simulink model "stewart_platform_final3"  (R2017a)
settings: Solver=ode45  StartTime=0.0  StopTime=40  MaxStep=0.2  RelTol=1e-3  EnableMultiTasking=on
model workspace (MAT data in the model file):
  g_density = 5
undefined symbols (not defined in the file): B, nom_length, P, X, Y, Z
libraries: nesl_utility x13, sm_stewart_platform_lib x8, sm_lib x7
(part 1 of 2)
Description:
  | Stewart Platform
  | 
  | This model shows a Stewart platform manipulator that can track a
  | parameterized reference trajectory. The shape, size, and kinematics of
  | the manipulator are highly configurable.
  | 
  | The reference trajectory is
  | specified in 6-D pose space, and an inverse kinematics module
  | converts it into one through 6-D leg position space.  A generic PID
  | controller attempts to drive the manipulator along the desired
  | trajectory.
  | 
  | 
  | Copyright 2011-2017 The MathWorks, Inc.
settings Model: FPTRunName=Active  Creator=MathWorks  LastModifiedBy=Omar
settings DataIOCC: LimitDataPoints=on  SaveFormat=Array  SignalLoggingSaveFormat=ModelDataLogs
settings OptimizationCC: ExpressionDepthLimit=2147483647  LifeSpan=inf
settings DebuggingCC: UnderspecifiedInitializationDetection=Classic  MergeDetectMultiDrivingBlocksExec=none  SolverPrmCheckMsg=warning  FcnCallInpInsideContextMsg=warning  StateNameClashWarn=warning  SFUnexpectedBacktrackingDiag=warning  SFNoUnconditionalDefaultTransitionDiag=warning  SFExecutionAtInitializationDiag=none
settings HardwareCC: ProdBitPerPointer=32  ProdBitPerSizeT=32  ProdBitPerPtrDiffT=32  ProdLargestAtomicFloat=None  ProdIntDivRoundTo=Undefined  ProdEndianess=Unspecified  ProdWordSize=32  ProdHWDeviceType=32-bit Generic
settings ModelReferenceCC: PropagateSignalLabelsOutOfModel=off
settings GRTTargetCC: TargetLangStandard=C89/C90 (ANSI)  GeneratePreprocessorConditionals=Disable all  CombineOutputUpdateFcns=off  GRTInterface=on
settings ConfigComp: CovMetricSettings=dw  CovHtmlReporting=on  CovSaveCumulativeToWorkspaceVar=on  CovSaveSingleToWorkspaceVar=on  CovExternalEMLEnable=off
settings SimscapeCC: SimscapeLogDataHistory=15000
settings ConfigurationSet: Description=SimMechanics 2G

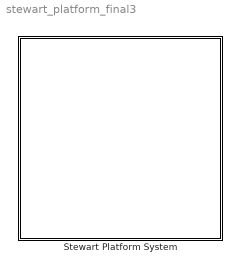
== system stewart_platform_final3 ==
  Stewart Platform System : Subsystem  mask(Stewart Platform System){base_rad=28, base_thick=8, platform_rad=18, platform_thick=2, hex_skew=-0.25, upper_leg_len=10, lower_leg_len=14, leg_rad=3, collar_thick=0.5, gripper_height=30, claw_length=8, claw_width=3, claw_thick=1, end_eff_base_thick=2, flange_len=3, flange_width=2.25, flange_thick=.8, ic_R=eye(3), ic_d=[0 0 71]', Kp=300, Ki=20, Kd=5}
      mask prompts: base_rad "Base Radius  (cm)"; base_thick "Base Thickness (cm)"; platform_rad "Platform Radius (cm)"; platform_thick "Platform Thickness (cm)"; hex_skew "Hexagon Skew"; upper_leg_len "Upper Leg Length (cm)"; lower_leg_len "Lower Leg Length (cm)"; leg_rad "Leg Radius (cm)"; collar_thick "Collar Thickness (cm)"; gripper_height "Gripper Height (cm)"; claw_length "Claw Length (cm)"; claw_width "Claw Width (cm)"; claw_thick "Claw Thickness (cm)"; end_eff_base_thick "Base Thickness (cm)"; flange_len "Flange Length (cm)"; flange_width "Flange Width (cm)"; flange_thick "Flange Thickness (cm)"; ic_R "Rotation Matrix [3 x 3]"; ic_d "Displacement Vector (cm) [3 x 1]"; Kp "Controller Proportional Gain (N / cm)"; Ki "Controller Integral Gain (N / (cm s))"; Kd "Controller Derivative Gain (N / (cm / s)))"
      mask help:
      | Models a complete Stewart platform manipulator system.  The system can be driven to position and orient a special gripper frame according to specified trajectories.
      |
      | The system comprises a mechanical manipulator, an inverse kinematics module, and a control system.
      mask init:
      | params = struct( ...
      |     'base_thick',        base_thick,     ...
      |     'base_radius',       base_rad,       ...
      |     'platform_thick',    platform_thick, ...
      |     'platform_radius',   platform_rad,   ...
      |     'skew',              hex_skew,       ...
      |     'flange_length',     flange_len,     ...
      |     'flange_width',      flange_width,   ...
      |     'flange_thick',      flange_thick,   ...
      |     'leg_radius',        leg_rad,        ...
      |     'upper_leg_length',  upper_leg_len,  ...
      |     'lower_leg_length',  lower_leg_len,  ...
      |     'gripper_height',    gripper_height  ...
      |     );
      | 
      | [B, P, nom_length] = sm_stewart_platform_setup(params);
      | 
      | lengths = sm_stewart_platform_ik(B, P, nom_length, ic_R, ic_d);
      mask Help:
      | A <em>Stewart Platform System</em> models a complete Stewart platform manipulator system.  The system can be driven to position and orient a special gripper frame according to specified trajectories.
      | 
      | <h3>Subsystems</h3>
      | 
      | A Stewart platform system comprises three primary subsystems:
      | 
      | <ol>
      | 
      | <li><b>Manipulator</b> The manipulator is the Simscape Multibody subsystem describing the mechanical structure of the Stewart platform.  The manipulator contains two hexagonal plates, a lower base plate and an upper platform plate, connected by six articulated legs.  The base plate is anchored to the world frame, and the platform plate is controlled to position and orient the gripper frame. The manipulator component provides sensing and actuation signals to interface to a controller.
      | 
      |   The manipulator is highly parameterized.  Most parameters of the Stewart platform system are physical lengths and other parameters that control the shapes and sizes of the components of the manipulator. By varying these parameters, a wide range of Stewart platform manipulators can be realized.
      | 
      | <li><b>Inverse Kinematics (IK) Module</b> The inverse kinematics module is a pure Simulink subsystem that maps time-varying signals describing the desired position and orientation of the gripper frame into time-varying scalar signals specifying the positions and velocities of the prismatic primitives of the leg joints.  This is an essential component of a complete Stewart platform system because the user of the system typically expresses a desired trajectory in the 6-D space of positions and orientations of the gripper frame, but the manipulator control is simplest in the 6-D space of leg joint positions. The IK module forms the bridge between these two spaces.
      | 
      |   The mathematics performed within the IK module is heavily dependent on the physical parameters that determine the shape and size of the manipulator itself.  Most of the parameters that govern the manipulator are also used within the IK module.
      | 
      | <li><b>Control System</b> The control system is a pure Simulink subsystem that attempts to drive the gripper frame along its desired trajectory by controlling the positions of the prismatic primitives of the leg joints. It uses a standard PID control scheme, with gains specified by Stewart platform system parameters.  The control uses no information about the forward or inverse kinematics of the platform; it simply tries to drive a point along a trajectory in 6-D space.
      | 
      |   The controller takes both the desired and actual leg position vectors and the first derivatives of these quantities.  It generates a 6-D commanded force output that can be used to drive the six leg lengths to thei desired values.
      | 
      |   Because the size and shape of the Stewart platform manipulator can vary significantly depending on the parameter settings, the controller gains may need to be adjusted in order to control the manipulator to the desired trajectory.
      | 
      | </ol>
      | 
      | <h3>Base and Platform Plates</h3>
      | 
      | The <em>Plates</em> tab parameters specify the geometry of the base and platform hexagon plates of the Stewart platform manipulator.  See the documentation of the <em>Hexagon Plate</em> library block for details.
      | 
      | <ul>
      | 
      | <li> <b>Base Radius</b> The radius of the base plate.  The vertices of the hexagonal cross section all lie on a circle of this radius.
      | 
      | <li> <b>Base Thickness</b> The thickness of the base plate.
      | 
      | <li> <b>Platform Radius</b> The radius of the platform plate.  The vertices of the hexagonal cross section all lie on a circle of this radius.
      | 
      | <li> <b>Platform Thickness</b> The thickness of the platform plate.
      | 
      | <li> <b>Hexagon Skew</b> The common skew factor of the base and platform plates. This value, in the range (-0.5, +0.5), determines the shape of the three-fold symmetric hexagons.  A zero skew factor produces regular hexagons.  As the skew factor magnitude increases, the hexagons become more triangular.
      | 
      | </ul>
      | 
      | <h3>Legs</h3>
      | 
      | The <em>Legs</em> tab parameters specify the common geometry of the six legs of the Stewart platform manipulator.  See the documentation of the <em>Leg</em> library block for details.
      | 
      | <ul>
      | 
      | <li> <b>Upper Leg Length</b> The length of the upper leg, including its end collars.
      | 
      | <li> <b>Lower Leg Length</b> The length of the lower leg, including its end collars.
      | 
      | <li> <b>Leg Radius</b> The common radius of the upper and lower leg segments. Each segment's cross section is a regular hexagon inscribed in a circle of this radius.
      | 
      | <li> <b>Collar Thickness</b> The thickness of the hexagonal collars adjoined to the ends of each leg segment.
      | 
      | </ul>
      | 
      | <h3>End Effector</h3>
      | 
      | The <em>End Eff</em> tab parameters specify the geometry of the end effector attached to the platform plate of the Stewart platform manipulator. See the documentation of the <em>End Effector</em> block within the <em>Manipulator</em> subsystem for details.
      | 
      | <ul>
      | 
      | <li> <b>Gripper Height</b> The vertical distance from the origin of the gripper frame to the top surface of the movable platform plate.
      | 
      | <li> <b>Claw Length</b> The length (height) of the trapezoidal claws of the gripper.
      | 
      | <li> <b>Claw Width</b> The width of the trapezoidal claws of the gripper where they attach to the gripper base.
      | 
      | <li> <b>Claw Thickness</b> The thickness of the trapezoidal claws of the gripper.
      | 
      | <li> <b>Base Thickness</b> The thickness of the triangular gripper base.
      | 
      | </ul>
      | 
      | <h3>Flanges</h3>
      | 
      | The <em>Flanges</em> tab parameters specify the common geometry of the 48 flanges attached to the hexagonal plates and legs of the Stewart platform manipulator.  Each of the 12 universal joints is supported by four flanges.  See the documentation of the <em>Flange</em> library block for details.
      | 
      | <ul>
      | 
      | <li> <b>Flange Length</b> The length of the rectangular prism portion of the flanges.
      | 
      | <li> <b>Flange Width</b> The width of the rectangular prism portion of the flanges.
      | 
      | <li> <b>Flange Thickness</b> The thickness of the flanges.
      | 
      | </ul>
      | 
      | <h3>Initial Conditions</h3>
      | 
      | The <em>IC</em> tab parameters specify the initial conditions of the Stewart Platform manipulator for simulation.  Specifically, these specify the <em>position</em> of the manipulator; the simulation always starts from a rest (zero velocity) state.
      | 
      | The initial position is defined by specifying pose of the gripper frame relative to the world frame.  This is typically a convenient parameterization for a user of the manipulator.  The world frame is also the reference frame of the manipulator base plate.  This is a frame with origin at the center of the manipulator base (which is in its interior), and with z-axis pointed directly upward.
      | 
      | An Update Diagram (Ctrl-D) operation will attempt to assemble the manipulator in the specified initial position.  Some initial positions may be incompatible with the kinematics of the manipulator, based on other parameter settings.  In such cases, the assembly will fail.
      | 
      | Also note that if the initial position differs significantly from the desired trajectory (specified through the input signal ports) at time zero, the manipulator's motion may be subject to large transients at the start of simulation.
      | 
      | <ul>
      | 
      | <li> <b>Rotation Matrix</b> The rotation matrix mapping directions in the gripper frame to directions in the world frame.  This should be a 3 x 3 orthogonal matrix determinant +1.  The columns of this matrix are the canonical i, j, and k unit vectors of the gripper frame resolved in world frame coordinates.
      | 
      | <li> <b>Displacement Vector</b> The location of the origin of the gripper frame in world frame coordinates.  This should be a 3 x 1 column vector.  The z-coordinate should generally be positive, on the order of the nominal lengths of the legs.
      | 
      | </ul>
      | 
      | If the rotation matrix is the identity and the x- and y-coordinates of the displacement vector are zero, the initial configuration of the manipulator will be symmetric with all leg positions equal.
      | 
      | <h3>Controller Gains</h3>
      | 
      | The <em>Control</em> tab parameters specify the gains of the internal controller used to control the manipulator's pose according to a specified trajectory.  The controller uses a generic PID control scheme.  The gains may need to be adjusted to be appropriate if the parameters governing the size and kinematics of the manipulator are changed significantly.
      | 
      | See the documentation of the <em>Controller</em> subsystem for details.
      | 
      | <ul>
      | 
      | <li> <b>Controller Proportional Gain</b> The proportional (P) gain of the internal PID controller.
      | 
      | <li> <b>Controller Integral Gain</b> The integral (I) gain of the internal PID controller.
      | 
      | <li> <b>Controller Derivative Gain</b> The derivative (D) gain of the internal PID controller.
      | 
      | </ul>
      | 
      | 
      | 
      | <h3>Ports</h3>
      | 
      | <ul>
      | 
      | <li><b>d</b> The desired displacement vector of the gripper frame relative to the world frame as a signal input.  This value should be a 3 x 1 vector in units of centimeters.  It specifies the desired origin of the gripper frame in world frame coordinates as a function of time.  This signal is analogous to the <em>Displacement Vector</em> on the <em>IC</em> parameter tab.
      | 
      | <li><b>R</b> The desired rotation matrix from the gripper frame to the world frame as a signal input.  This value should be a 3 x 3 orthogonal matrix with +1 determinant.  The columns of this matrix are the canonical i, j, and k unit vectors of the gripper frame resolved in world frame coordinates, specified as functions of time.  This signal is analogous to the <em>Rotation Matrix</em> on the <em>IC</em> parameter tab.
      | 
      | <li><b>d'</b> The first time derivative of the desired displacement vector of the gripper frame relative to the world frame as a signal input.  This value should be the first time derivative of the signal provided on the <em>d</em> port: a 3 x 1 vector in units of centimeters/second. It specifies the velocity of the origin of the gripper frame in  world frame coordinates as a function of time.
      | 
      | <li><b>R'</b> The first time derivative of the desired rotation matrix from the gripper frame to the world frame as a signal input.  This value should be the first time derivative of the signal provided on the <em>R</em> port: a 3 x 3 matrix.
      | 
      | <li><b>Pos</b> The position of the gripper with respect to the world frame as a 3 x 1 position vector in units of centimeters.
      | </ul>
      | 
      | <!--  LocalWords:  Eff IC Ctrl IK
      |  -->
      mask Display:
      | image(imread('StewPlatBlock.png'))
      | color('yellow')
      | port_label('Input', 1, 'd')
      | port_label('Input', 2, 'R')
      | port_label('Input', 3, 'd''')
      | port_label('Input', 4, 'R''')
      | port_label('Output', 1, 'Pos')

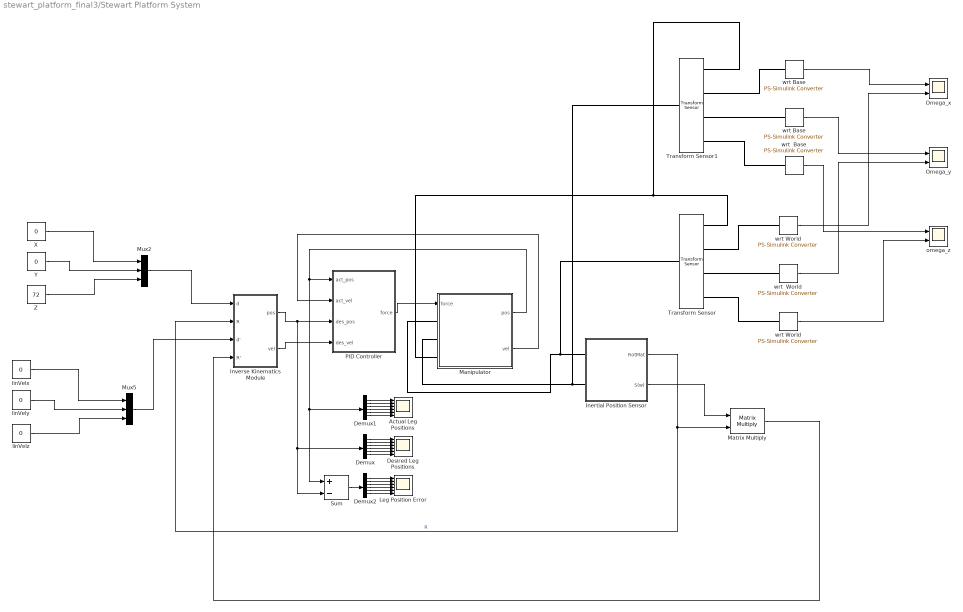
== system stewart_platform_final3/Stewart Platform System ==
  " wrt World" : nesl_utility/PS-Simulink Converter  PhysicalDomain=network_engine_domain  SubClassName=ps_output  LeftPortType=input  RightPortType=output  PseudoPeriodic=off  Frequencies=[]  Unit=1  AffineConversion=off
  Actual Leg Positions : Scope  NumInputPorts=6
  Demux : Demux  Outputs=6
  Demux1 : Demux  Outputs=6
  Demux2 : Demux  Outputs=6
  Desired Leg Positions : Scope  NumInputPorts=6
  Inertial Position Sensor : Subsystem
  Inverse Kinematics Module : Subsystem  mask(Stewart Platform Inverse Kinematics){}
      mask help:
      | Performs the essential inverse kinematic computations for a Stewart platform manipulator.
      |
      | Given a desired dynamic state of a Stewart platform manipulator specified by a 3-D rigid transformation from the gripper frame to the base reference frame, and the first time derivative of this transformation, this block computes the positions and velocities of the prismatic primitives of the six cylindrical leg joints necessary to achieve the desired dynamic state.
      mask Help:
      | A <em>Stewart Platform Inverse Kinematics</em> performs the essential inverse kinematic computations for a Stewart platform manipulator.
      | 
      | Given a desired dynamic state of a Stewart platform manipulator specified by a 3-D rigid transformation from the gripper frame to the base reference frame, and the first time derivative of this transformation, this block computes the positions and velocities of the prismatic primitives of the six cylindrical leg joints necessary to achieve the desired dynamic state.
      | 
      | <h3>Manipulator Transformation</h3>
      | 
      | The desired dynamic state of a Stewart platform manipulator may be specified by a single 3-D rigid transformation, called the <em>manipulator transformation</em>, and its time derivative.  The transformation is from <em>gripper</em> frame to <em>base</em> frame coordinates.  The base frame is attached to the base plate of the manipulator.  Its origin is located at the center of the base, and the z-axis points directly upward.  The gripper frame is located somewhere directly above the center of platform plate of the manipulator, and is aligned with the base frame when the positions of the prismatic primitives of all six cylindrical leg joints are equal.
      | 
      | In the following discussions, let <b>R</b> and <b>d</b> specify the rotation matrix and displacement vector, respectively, of the manipulator transformation. That is, <b>d</b> is the origin of the gripper frame specified in base frame coordinates, and the columns of <b>R</b> are the canonical <b>i</b>, <b>j</b>, and <b>k</b> vectors of the gripper frame resolved in base frame coordinates.
      | Let <b>R'</b> and <b>d'</b> be the first time derivatives of <b>R</b> and <b>d</b>, respectively.
      | 
      | <h3>Inverse Kinematics</h3>
      | 
      | Each of the six legs of the manipulator is attached between a pair of universal joints: one on the base plate and one on the platform plate.  Each leg has an internal knee joint with a sensed and actuated prismatic primitive.
      | Let <em>q_i</em> and <em>q_i'</em> be the position and velocity of this primitive on Leg <em>i</em>.  Let <em>L0</em> denote the <em>nominal</em> lengths of the legs.  This is the length of a leg when its prismatic primitive is at the zero position.
      | 
      | The goal of the inverse kinematics computation is to determine the values of <em>q_i</em> and <em>q_i'</em> for i = 1, ..., 6 needed to achieve a particular manipulator transformation and its derivative.
      | 
      | The key to understanding the inverse kinematics computations is to consider the positions of the centers of the pairs of universal joints.  (These points are the centers of the crosspieces visible in the visualization of the manipulator.)
      | 
      | Let <b>b</b>_i and <b>p</b>_i be the 3-D points specifying the center of the universal joints on the base and platform plates, respectively, to which Leg <em>i</em> is connected. <b>b</b>_i is specified in base frame coordinates, and <b>p</b>_i is specified in gripper frame coordinates.  Then the desired position of the prismatic primitive of the knee joint of Leg <em>i</em> is given by
      | 
      | <em>q_i</em> = || <b>R</b> <b>p</b>_i + <b>d</b> - <b>b</b>_i || - <em>L0</em>.
      | 
      | Denote the vector within the norm expression above as <b>o</b>_i (<b>o</b> for <em>offset</em>).
      | 
      | The desired velocity of the prismatic primitive of the knee joint of Leg <em>i</em> is obtained by differentiating the expression for <em>q_i</em>. Noting that <b>p</b>_i, <b>b</b>_i, and <em>L0</em> are constant, the result is:
      | 
      | <em>q_i'</em> = [ (<b>R'</b> <b>p</b>_i + <b>d'</b>) . <b>o</b>_i ] / || <b>o</b>_i ||.
      | 
      | Note that the denominator of this expression is equal to the vector norm in the expression for <em>q_i</em>.
      | 
      | This block computes the values of all six prismatic primitive positions and velocities according to the expressions above.  The computation of the (constant) <b>p</b>_i and <b>b</b>_i points is highly dependent on the manipulator kinematics and done in the mask initialization of the containing <em>Stewart Platform System</em> block.
      | 
      | <h3>Ports</h3>
      | 
      | <ul>
      | 
      | <li> <b>d</b> The displacement vector of the desired manipulator transformation (see above) in units of centimeters.
      | 
      | <li> <b>R</b> The rotation matrix of the desired manipulator transformation (see above).
      | 
      | <li> <b>d'</b> The time derivative of the displacement vector of the desired manipulator transformation in units of centimeters/second.
      | 
      | <li> <b>R'</b> The time derivative of the rotation matrix of the desired manipulator transformation.
      | 
      | <li> <b>pos</b> The computed positions of the prismatic primitives of the six leg joints, as a 6 x 1 vector in units of centimeters.
      | 
      | <li> <b>vel</b> The computed velocities of the prismatic primitives of the six leg joints, as a 6 x 1 vector in units of centimeters/second.
      | 
      | 
      | </ul>
      | 
      | <!--  LocalWords:  ith pos vel
      |  -->
  Leg Position Error : Scope  NumInputPorts=6
  Manipulator : Subsystem  mask(Stewart Platform Manipulator){}
      mask help: Models the mechanical portion of a complete Stewart platform manipulator system: the manipulator itself. Almost all of the Simscape Multibody blocks of the full system are contained in the manipulator subsystem.
      mask Help:
      | A <em>Stewart Platform Manipulator</em> models the mechanical portion of a complete Stewart platform manipulator system: the manipulator itself.  Almost all of the Simscape Multibody blocks of the full system are contained in the manipulator subsystem.
      | 
      | The manipulator subsystem exposes two frames: the world frame, to which the base is anchored, and the gripper frame, which is the frame at the distil end of the end effector.  Typically, a user wants to control the manipulator transformation, which is the 3-D rigid transformation from the gripper frame to the world frame.
      | 
      | The manipulator subsystem has no internal control.  However, it reports the positions and velocities of the prismatic primitives of all six cylindrical leg joints as output signals and takes the actuation forces to be applied to these primitives as input signals.  When connected to an appropriate controller, these signals are sufficient to provide any of a variety of control schemes for the manipulator.
      | 
      | <h3>Parameterization</h3>
      | 
      | The manipulator is highly parameterized.  Most of the physical dimensions of its component pieces can be controlled via parameters.  These parameters are all defined in the containing <em>Stewart Platform System</em>.  The manipulator's parameters are inherited from that block; they are not defined explicitly in this block's mask.  The parameters are also needed for the <em>Stewart Platform Inverse Kinematics</em> block.
      | 
      | See the documentation of the <em>Stewart Platform System</em> block for details.
      | 
      | <h3>Ports</h3>
      | 
      | <ul>
      | 
      | <li> <b>gripper</b> The gripper frame.  This frame is fixed at the distil end of the end effector attached to the platform plate of the Stewart platform manipulator.  It is identified with a frame glyph in the visualization of the manipulator.  Typically, a user of the manipulator wants to control the pose of this frame, with respect to a reference frame such as world.
      | 
      | <li> <b>world</b> The world frame.  This is also the reference frame of the base plate of the Stewart platform manipulator, which is rigidly attached to the world frame.
      | 
      | <li><b>pos</b> The positions of the prismatic primitives of the six leg joints as a 6 x 1 output signal in units of centimeters.
      | 
      | <li><b>vel</b> The velocities of the prismatic primitives of the six leg joints as a 6 x 1 output signal in units of centimeters/second.
      | 
      | <li><b>force</b> The actuation forces applied to the prismatic primitives of the six leg joints as a 6 x 1 input signal in units of Newtons.
      | 
      | </ul>
      | 
      | <!--  LocalWords:  Eff IC Ctrl pos vel
      |  -->
      mask Display:
      | image(imread('StewPlat.png'))
      | color('white')
      | port_label('LConn', 1, 'World')
      | port_label('LConn', 2, 'Base')
      | port_label('LConn', 3, 'Top')
      | color('yellow')
      | port_label('Input', 1, 'force')
      | port_label('Output', 1, 'pos')
      | port_label('Output', 2, 'vel')
  Matrix Multiply : Product  Multiplication=Matrix(*)
  Mux2 : Mux  Inputs=3
  Mux5 : Mux  Inputs=3
  Omega_x : Scope  NumInputPorts=2
  Omega_y : Scope  NumInputPorts=2
  PID Controller : Subsystem  mask(PID Controller){Kp=Kp, Ki=Ki, Kd=Kd}
      mask prompts: Kp "Proportional Gain"; Ki "Integral Gain"; Kd "Derivative Gain"
      mask help:
      | Generates an actuation output based on a desired trajectory and an actual trajectory, using a generic proportional-integral-derivative (PID) control law.  The three control gains are specified through parameters.
      |
      | Both the desired and actual trajectories are specified by separate position and velocity input signals.  The controller is generic and can control to trajectories through state spaces of arbitrary dimension; the only requirement is that all four inputs have the same dimension.
      mask Help:
      | A <em>PID Controller</em> generates an actuation output based on a desired trajectory and an actual trajectory, using a generic proportional-integral-derivative (PID) control law.  The three control gains are specified through parameters.
      | 
      | Both the desired and actual trajectories are specified by separate position and velocity input signals.  The controller is generic and can control to trajectories through state spaces of arbitrary dimension; the only requirement is that all four inputs have the same dimension.
      | 
      | This block is not specific to the Stewart platform and could serve in any general purpose control library.  For the Stewart platform application, the trajectories are all through the 6-D leg-position space.
      | 
      | <h3>Gains</h3>
      | 
      | The parameters specify the gains of the controller.
      | 
      | <ul>
      | 
      | <li> <b>Proportional Gain</b> The gain that determines the strength of the control actuation in response to current deviations between actual and desired positions.  This affects the responsiveness of the controller but can lead to instability if set too high.
      | 
      | <li> <b>Integral Gain</b> The gain that determines the strength of the control actuation in response to deviations between actual and desired positions that persist over time.  A nonzero integral term is often necessary to avoid <em>droop</em> (steady-state error).  Higher values reduce the transient response of the controller but can cause overshoot in the controlled position.
      | 
      | <li> <b>Derivative Gain</b> The gain that determines the strength of the control actuation in response to the derivative of the deviations between actual and desired positions.  This is a damping component used to reduce overshoot in the controlled position; the tradeoff is that it reduces the transient response of the controller.  Higher values increase the stiffness of the system and can lead to instability.
      | 
      | </ul>
      | 
      | 
      | <h3>Ports</h3>
      | 
      | <ul>
      | 
      | <li> <b>act_pos</b> The current actual position of the plant.
      | 
      | <li> <b>act_pos</b> The current actual velocity of the plant.  This should be the time derivative of the <em>act_pos</em> signal.
      | 
      | <li> <b>des_pos</b> The current desired position of the plant.
      | 
      | <li> <b>des_pos</b> The current desired velocity of the plant.  This should be the time derivative of the <em>des_pos</em> signal.
      | 
      | </ul>
  Sum : Sum  Inputs=+-
  Transform Sensor : sm_lib/Frames and Transforms/Transform Sensor  MeasurementFrame=World  SenseAngle=off  SenseAxis=off  SenseAngle1=off  SenseAngle2=off  SenseAngle3=off  SenseQ=off  SenseR=off  SenseOmegaX=on  SenseOmegaY=on  SenseOmegaZ=on  SenseOmega1=off  SenseOmega2=off  SenseOmega3=off  SenseQDot=off  SenseRDot=off  SenseAlphaX=off  SenseAlphaY=off  SenseAlphaZ=off  SenseAlpha1=off  SenseAlpha2=off  SenseAlpha3=off  SenseQDDot=off  SenseRDDot=off  SenseX=off  SenseY=off  SenseZ=off  SenseRad=off  SenseAzim=off  SenseDist=off  SenseInc=off  SenseXDot=off  SenseYDot=off  SenseZDot=off  SenseRadDot=off  SenseAzimDot=off  SenseDistDot=off  SenseIncDot=off  SenseXDDot=off  SenseYDDot=off  SenseZDDot=off  SenseRadDDot=off  SenseAzimDDot=off  SenseDistDDot=off  SenseIncDDot=off
  Transform Sensor1 : sm_lib/Frames and Transforms/Transform Sensor  MeasurementFrame=World  SenseAngle=off  SenseAxis=off  SenseAngle1=off  SenseAngle2=off  SenseAngle3=off  SenseQ=off  SenseR=off  SenseOmegaX=on  SenseOmegaY=on  SenseOmegaZ=on  SenseOmega1=off  SenseOmega2=off  SenseOmega3=off  SenseQDot=off  SenseRDot=off  SenseAlphaX=off  SenseAlphaY=off  SenseAlphaZ=off  SenseAlpha1=off  SenseAlpha2=off  SenseAlpha3=off  SenseQDDot=off  SenseRDDot=off  SenseX=off  SenseY=off  SenseZ=off  SenseRad=off  SenseAzim=off  SenseDist=off  SenseInc=off  SenseXDot=off  SenseYDot=off  SenseZDot=off  SenseRadDot=off  SenseAzimDot=off  SenseDistDot=off  SenseIncDot=off  SenseXDDot=off  SenseYDDot=off  SenseZDDot=off  SenseRadDDot=off  SenseAzimDDot=off  SenseDistDDot=off  SenseIncDDot=off
  X : Constant  Value=0
  Y : Constant  Value=0
  Z : Constant  Value=72
  linVelx : Constant  Value=0
  linVely : Constant  Value=0
  linVelz : Constant  Value=0
  omega_z : Scope  NumInputPorts=2
  "wrt  Base " : nesl_utility/PS-Simulink Converter  PhysicalDomain=network_engine_domain  SubClassName=ps_output  LeftPortType=input  RightPortType=output  PseudoPeriodic=off  Frequencies=[]  Unit=1  AffineConversion=off
  wrt  World : nesl_utility/PS-Simulink Converter  PhysicalDomain=network_engine_domain  SubClassName=ps_output  LeftPortType=input  RightPortType=output  PseudoPeriodic=off  Frequencies=[]  Unit=1  AffineConversion=off
  "wrt Base " : nesl_utility/PS-Simulink Converter  PhysicalDomain=network_engine_domain  SubClassName=ps_output  LeftPortType=input  RightPortType=output  PseudoPeriodic=off  Frequencies=[]  Unit=1  AffineConversion=off
  "wrt Base " : nesl_utility/PS-Simulink Converter  PhysicalDomain=network_engine_domain  SubClassName=ps_output  LeftPortType=input  RightPortType=output  PseudoPeriodic=off  Frequencies=[]  Unit=1  AffineConversion=off
  wrt World : nesl_utility/PS-Simulink Converter  PhysicalDomain=network_engine_domain  SubClassName=ps_output  LeftPortType=input  RightPortType=output  PseudoPeriodic=off  Frequencies=[]  Unit=1  AffineConversion=off
  wires:
  Manipulator/2(vel) -> PID Controller/2(act_vel)
  Demux/1 -> Desired Leg Positions/1
  Demux/2 -> Desired Leg Positions/2
  Demux/3 -> Desired Leg Positions/3
  Demux/4 -> Desired Leg Positions/4
  Demux/5 -> Desired Leg Positions/5
  Demux/6 -> Desired Leg Positions/6
  Demux1/1 -> Actual Leg Positions/1
  Demux1/2 -> Actual Leg Positions/2
  Demux1/3 -> Actual Leg Positions/3
  Demux1/4 -> Actual Leg Positions/4
  Demux1/5 -> Actual Leg Positions/5
  Demux1/6 -> Actual Leg Positions/6
  Demux2/1 -> Leg Position Error/1
  Demux2/2 -> Leg Position Error/2
  Demux2/3 -> Leg Position Error/3
  Demux2/4 -> Leg Position Error/4
  Demux2/5 -> Leg Position Error/5
  Demux2/6 -> Leg Position Error/6
  Sum/1 -> Demux2/1
  PID Controller/1(force) -> Manipulator/1(force)
  Manipulator/1(pos) -> PID Controller/1(act_pos), Demux1/1, Sum/1
  Inverse Kinematics Module/2(vel) -> PID Controller/4(des_vel)
  Inverse Kinematics Module/1(pos) -> PID Controller/3(des_pos), Sum/2, Demux/1
  Inertial Position Sensor/1(RotMat) -> Matrix Multiply/2, Inverse Kinematics Module/2(R)  "R"
  X/1 -> Mux2/1
  Y/1 -> Mux2/2
  Z/1 -> Mux2/3
  Mux2/1 -> Inverse Kinematics Module/1(d)
  linVelz/1 -> Mux5/3
  linVely/1 -> Mux5/2
  linVelx/1 -> Mux5/1
  Mux5/1 -> Inverse Kinematics Module/3(d')
  Inertial Position Sensor/2("S(w) ") -> Matrix Multiply/1
  Matrix Multiply/1 -> Inverse Kinematics Module/4(R')
  "wrt Base "/1 -> Omega_x/1
  wrt World/1 -> Omega_x/2
  "wrt Base "/1 -> Omega_y/1
  wrt  World/1 -> Omega_y/2
  "wrt  Base "/1 -> omega_z/1
  " wrt World"/1 -> omega_z/2
  connections:
  Manipulator/LConn2 -- Transform Sensor1/LConn1 -- Inertial Position Sensor/LConn2
  Manipulator/LConn1 -- Inertial Position Sensor/LConn1 -- Transform Sensor/LConn1
  Transform Sensor/RConn2 -- wrt World/LConn1
  Transform Sensor/RConn3 -- wrt  World/LConn1
  Transform Sensor/RConn4 -- " wrt World"/LConn1
  Manipulator/LConn3 -- Transform Sensor/RConn1 -- Transform Sensor1/RConn1
  "wrt Base "/LConn1 -- Transform Sensor1/RConn3
  "wrt  Base "/LConn1 -- Transform Sensor1/RConn4
  Transform Sensor1/RConn2 -- "wrt Base "/LConn1

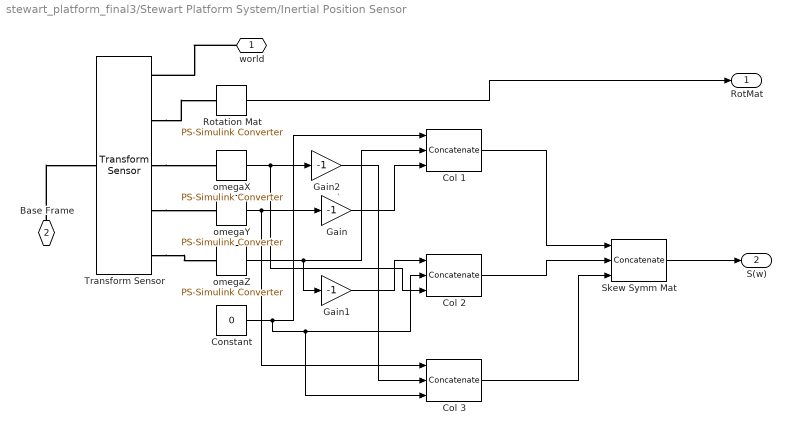
== system stewart_platform_final3/Stewart Platform System/Inertial Position Sensor ==
  note: `
  " omegaZ " : nesl_utility/PS-Simulink Converter  PhysicalDomain=network_engine_domain  SubClassName=ps_output  LeftPortType=input  RightPortType=output  PseudoPeriodic=off  Frequencies=[]  Unit=rad/s  AffineConversion=off
  Col 1 : Concatenate  NumInputs=3  Mode=Multidimensional array
  Col 2 : Concatenate  NumInputs=3  Mode=Multidimensional array
  Col 3 : Concatenate  NumInputs=3  Mode=Multidimensional array
  Constant : Constant  Value=0
  Gain : Gain  Gain=-1
  Gain1 : Gain  Gain=-1
  Gain2 : Gain  Gain=-1
  Rotation Mat : nesl_utility/PS-Simulink Converter  PhysicalDomain=network_engine_domain  SubClassName=ps_output  LeftPortType=input  RightPortType=output  PseudoPeriodic=off  Frequencies=[]  Unit=rad  AffineConversion=off
  Skew Symm Mat : Concatenate  NumInputs=3  Mode=Multidimensional array  ConcatenateDimension=2
  Transform Sensor : sm_lib/Frames and Transforms/Transform Sensor  MeasurementFrame=World  SenseAngle=off  SenseAxis=off  SenseAngle1=off  SenseAngle2=off  SenseAngle3=off  SenseQ=off  SenseR=on  SenseOmegaX=on  SenseOmegaY=on  SenseOmegaZ=on  SenseOmega1=off  SenseOmega2=off  SenseOmega3=off  SenseQDot=off  SenseRDot=off  SenseAlphaX=off  SenseAlphaY=off  SenseAlphaZ=off  SenseAlpha1=off  SenseAlpha2=off  SenseAlpha3=off  SenseQDDot=off  SenseRDDot=off  SenseX=off  SenseY=off  SenseZ=off  SenseRad=off  SenseAzim=off  SenseDist=off  SenseInc=off  SenseXDot=off  SenseYDot=off  SenseZDot=off  SenseRadDot=off  SenseAzimDot=off  SenseDistDot=off  SenseIncDot=off  SenseXDDot=off  SenseYDDot=off  SenseZDDot=off  SenseRadDDot=off  SenseAzimDDot=off  SenseDistDDot=off  SenseIncDDot=off
  omegaX : nesl_utility/PS-Simulink Converter  PhysicalDomain=network_engine_domain  SubClassName=ps_output  LeftPortType=input  RightPortType=output  PseudoPeriodic=off  Frequencies=[]  Unit=rad/s  AffineConversion=off
  omegaY : nesl_utility/PS-Simulink Converter  PhysicalDomain=network_engine_domain  SubClassName=ps_output  LeftPortType=input  RightPortType=output  PseudoPeriodic=off  Frequencies=[]  Unit=rad/s  AffineConversion=off
  world : PMIOPort  Port=1  Side=Left
  Base Frame : PMIOPort  Port=2  Side=Left
  RotMat : Outport
  "S(w) " : Outport  Port=2
  wires:
  Rotation Mat/1 -> RotMat/1
  Constant/1 -> Col 3/3, Col 2/2, Col 1/1
  " omegaZ "/1 -> Gain1/1, Col 1/2
  omegaY/1 -> Col 3/1, Gain/1
  Gain/1 -> Col 1/3
  Gain1/1 -> Col 2/1
  omegaX/1 -> Gain2/1, Col 2/3
  Gain2/1 -> Col 3/2
  Col 1/1 -> Skew Symm Mat/1
  Col 2/1 -> Skew Symm Mat/2
  Col 3/1 -> Skew Symm Mat/3
  Skew Symm Mat/1 -> "S(w) "/1
  connections:
  Transform Sensor/RConn2 -- Rotation Mat/LConn1
  Transform Sensor/RConn3 -- omegaX/LConn1
  Transform Sensor/RConn4 -- omegaY/LConn1
  Transform Sensor/RConn5 -- " omegaZ "/LConn1
  world/RConn1 -- Transform Sensor/RConn1
  Base Frame/RConn1 -- Transform Sensor/LConn1

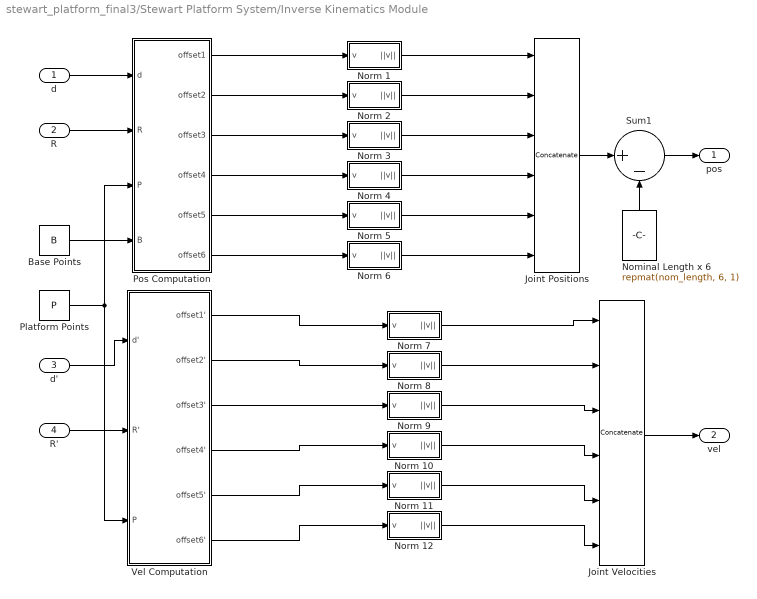
== system stewart_platform_final3/Stewart Platform System/Inverse Kinematics Module ==
  d : Inport
  R : Inport  Port=2
  d' : Inport  Port=3
  R' : Inport  Port=4
  Base Points : Constant  Value=B
  Joint Positions : Concatenate  NumInputs=6  Mode=Multidimensional array
  Joint Velocities : Concatenate  NumInputs=6  Mode=Multidimensional array
  Nominal Length x 6 : Constant  Value=repmat(nom_length, 6, 1)
  Norm 1 : Subsystem
  Norm 10 : Subsystem
  Norm 11 : Subsystem
  Norm 12 : Subsystem
  Norm 2 : Subsystem
  Norm 3 : Subsystem
  Norm 4 : Subsystem
  Norm 5 : Subsystem
  Norm 6 : Subsystem
  Norm 7 : Subsystem
  Norm 8 : Subsystem
  Norm 9 : Subsystem
  Platform Points : Constant  Value=P
  Pos Computation : Subsystem
  Sum1 : Sum  Inputs=|+-
  Vel Computation : Subsystem
  pos : Outport
  vel : Outport  Port=2
  wires:
  Joint Positions/1 -> Sum1/1
  Nominal Length x 6/1 -> Sum1/2
  Sum1/1 -> pos/1
  d/1 -> Pos Computation/1(d)
  R/1 -> Pos Computation/2(R)
  Base Points/1 -> Pos Computation/4(B)
  Platform Points/1 -> Vel Computation/3(P), Pos Computation/3(P)
  Pos Computation/4(offset4) -> Norm 4/1(v)
  Pos Computation/3(offset3) -> Norm 3/1(v)
  Pos Computation/2(offset2) -> Norm 2/1(v)
  Pos Computation/1(offset1) -> Norm 1/1(v)
  Pos Computation/5(offset5) -> Norm 5/1(v)
  Pos Computation/6(offset6) -> Norm 6/1(v)
  Norm 1/1(||v||) -> Joint Positions/1
  Norm 6/1(||v||) -> Joint Positions/6
  Norm 2/1(||v||) -> Joint Positions/2
  Norm 3/1(||v||) -> Joint Positions/3
  Norm 4/1(||v||) -> Joint Positions/4
  Norm 5/1(||v||) -> Joint Positions/5
  d'/1 -> Vel Computation/1(d')
  Joint Velocities/1 -> vel/1
  R'/1 -> Vel Computation/2(R')
  Norm 11/1(||v||) -> Joint Velocities/5
  Norm 10/1(||v||) -> Joint Velocities/4
  Norm 9/1(||v||) -> Joint Velocities/3
  Norm 8/1(||v||) -> Joint Velocities/2
  Norm 12/1(||v||) -> Joint Velocities/6
  Norm 7/1(||v||) -> Joint Velocities/1
  Vel Computation/6(offset6') -> Norm 12/1(v)
  Vel Computation/5(offset5') -> Norm 11/1(v)
  Vel Computation/1(offset1') -> Norm 7/1(v)
  Vel Computation/2(offset2') -> Norm 8/1(v)
  Vel Computation/3(offset3') -> Norm 9/1(v)
  Vel Computation/4(offset4') -> Norm 10/1(v)

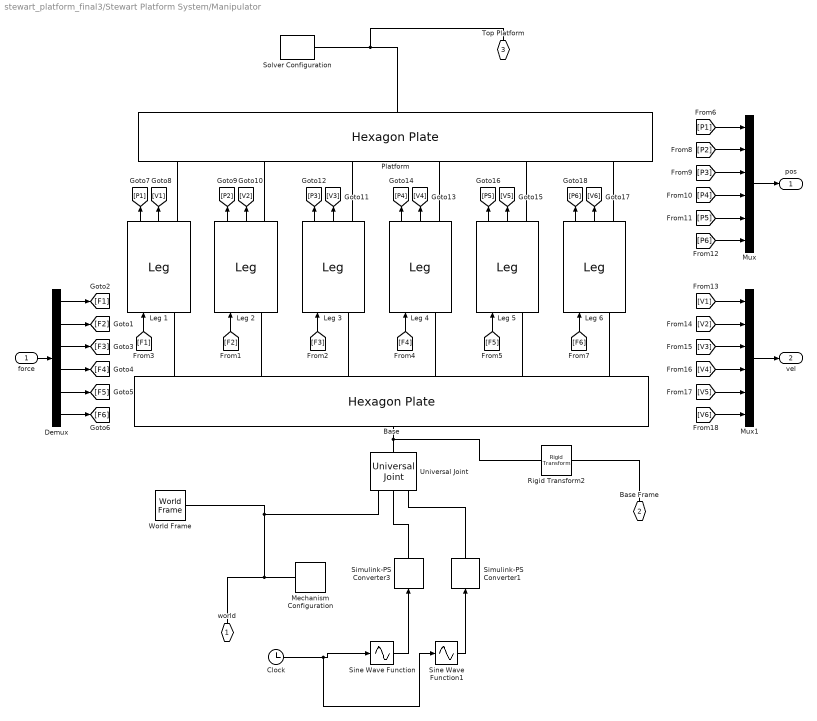
== system stewart_platform_final3/Stewart Platform System/Manipulator ==
  force : Inport
  Base : sm_stewart_platform_lib/Hexagon Plate  kind=base  hex_rad=base_rad  hex_thick=base_thick  hex_skew=hex_skew  flange_sep=2 * leg_rad * cos(pi/6) - flange_thick  flange_len=flange_len  flange_width=flange_width  flange_thick=flange_thick  diffuse=[0.4 0.3 0.2 0.5]  specular=[0 0 0]  shininess=10
  Clock : Clock
  Demux : Demux  Outputs=6
  Leg 1 : sm_stewart_platform_lib/Leg  upper_leg_len=upper_leg_len  lower_leg_len=lower_leg_len  rad=leg_rad  collar_thick=collar_thick  flange_len=flange_len  flange_width=flange_width  flange_thick=flange_thick  asm_offset=lengths(1)
  Leg 2 : sm_stewart_platform_lib/Leg  upper_leg_len=upper_leg_len  lower_leg_len=lower_leg_len  rad=leg_rad  collar_thick=collar_thick  flange_len=flange_len  flange_width=flange_width  flange_thick=flange_thick  asm_offset=lengths(2)
  Leg 3 : sm_stewart_platform_lib/Leg  upper_leg_len=upper_leg_len  lower_leg_len=lower_leg_len  rad=leg_rad  collar_thick=collar_thick  flange_len=flange_len  flange_width=flange_width  flange_thick=flange_thick  asm_offset=lengths(3)
  Leg 4 : sm_stewart_platform_lib/Leg  upper_leg_len=upper_leg_len  lower_leg_len=lower_leg_len  rad=leg_rad  collar_thick=collar_thick  flange_len=flange_len  flange_width=flange_width  flange_thick=flange_thick  asm_offset=lengths(4)
  Leg 5 : sm_stewart_platform_lib/Leg  upper_leg_len=upper_leg_len  lower_leg_len=lower_leg_len  rad=leg_rad  collar_thick=collar_thick  flange_len=flange_len  flange_width=flange_width  flange_thick=flange_thick  asm_offset=lengths(5)
  Leg 6 : sm_stewart_platform_lib/Leg  upper_leg_len=upper_leg_len  lower_leg_len=lower_leg_len  rad=leg_rad  collar_thick=collar_thick  flange_len=flange_len  flange_width=flange_width  flange_thick=flange_thick  asm_offset=lengths(6)
  Mechanism Configuration : sm_lib/Utilities/Mechanism Configuration  UniformGravity=Constant  GravityVector=[0 0 -9.81]  GravityUnits=m/s^2  LinearizationDelta=0.001
  Mux : Mux  Inputs=6
  Mux1 : Mux  Inputs=6
  Platform : sm_stewart_platform_lib/Hexagon Plate  kind=platform  hex_rad=platform_rad  hex_thick=platform_thick  hex_skew=hex_skew  flange_sep=2 * leg_rad * cos(pi/6) - flange_thick  flange_len=flange_len  flange_width=flange_width  flange_thick=flange_thick  diffuse=[.7 .7 .3 0.75]  specular=[.7 .7 .3 0.75]  shininess=90
  Rigid Transform2 : sm_lib/Frames and Transforms/Rigid Transform  TranslationMethod=StandardAxis  TranslationStandardOffset=.05  TranslationLengthUnit=m  TranslationStandardAxis=+Z  TranslationCartesianOffset=[0 0 0]  TranslationROffset=0  TranslationROffsetUnits=m  TranslationZOffset=0  TranslationZOffsetUnits=m  TranslationThetaOffset=0  TranslationThetaOffsetUnits=deg  RotationMethod=RotationMatrix  RotationAngleUnits=deg  RotationStandardAxis=+Z  RotationAngle=0.0  RotationArbitraryAxis=[0 0 1]  FollAlignAxisA=+X  BaseAlignAxisA=+Y  FollAlignAxisB=+Y  BaseAlignAxisB=+Z  RotationSequenceAxes=FollowerAxes  RotationSequence=XYX  RotationSequenceAngles=[0 0 0]  RotationSequenceAnglesUnits=deg  RotationMatrix=[1 0 0; 0 1 0; 0 0 1]
  Simulink-PS Converter1 : nesl_utility/Simulink-PS Converter  PhysicalDomain=network_engine_domain  SubClassName=ps_input  LeftPortType=input  RightPortType=output  PseudoPeriodic=off  Frequencies=[]  NoiseDistribution=none  NoiseParameters=[]  Unit=1  AffineConversion=off  FilteringAndDerivatives=filter  SimscapeFilterOrder=2  InputFilterTimeConstant=0.1  UdotUserProvided=2
  Simulink-PS Converter3 : nesl_utility/Simulink-PS Converter  PhysicalDomain=network_engine_domain  SubClassName=ps_input  LeftPortType=input  RightPortType=output  PseudoPeriodic=off  Frequencies=[]  NoiseDistribution=none  NoiseParameters=[]  Unit=1  AffineConversion=off  FilteringAndDerivatives=filter  SimscapeFilterOrder=2  InputFilterTimeConstant=0.1  UdotUserProvided=2
  Sine Wave Function : Sin  TimeSource=Use external signal  Amplitude=0.15  SampleTime=0
  Sine Wave Function1 : Sin  TimeSource=Use external signal  Amplitude=0.15  SampleTime=0
  Solver Configuration : nesl_utility/Solver Configuration  PhysicalDomain=network_engine_domain  SubClassName=solver  LeftPortType=input  RightPortType=generic  Accelerate=off  Tones=[]  Harmonics=[]  SimulateNoise=off  Profile=off  UseLocalSampling=off  EnableSwitchedLinearOptims=on  FrequencyDomain=off  UseCCode=off  RelTol=0.001  AbsTol=1e-06  MinStep=1e-09  ToWorkspace=off  RevertToSquareIcSolve=off  NumHomotopyIterations=100  PhasorMode=off  PhasorModeNumHarmonics=1  OverrideAbsTol=off  DoDC=off  ResidualTolerance=1e-9  UseLocalSolver=off  LocalSolverChoice=NE_BACKWARD_EULER_ADVANCER  LocalSolverSampleTime=.001  DoFixedCost=off  MaxNonlinIter=3  MaxModeIter=2  LinearAlgebra=Sparse  DelaysMemoryBudget=1024  AutomaticFiltering=on  FilteringTimeConstant=0.001
  Universal Joint : sm_lib/Joints/Universal Joint  SenseConstraintForce=off  SenseConstraintForceX=off  SenseConstraintForceY=off  SenseConstraintForceZ=off  SenseConstraintTorque=off  SenseConstraintTorqueX=off  SenseConstraintTorqueY=off  SenseConstraintTorqueZ=off  SenseTotalForce=off  SenseTotalForceX=off  SenseTotalForceY=off  SenseTotalForceZ=off  SenseTotalTorque=off  SenseTotalTorqueX=off  SenseTotalTorqueY=off  SenseTotalTorqueZ=off  CompositeWrenchDir=FollowerOnBase  CompositeWrenchFrame=BaseFrame  RxEquilibriumPosition=0  RxEquilibriumPositionUnits=deg  RxSpringStiffness=0  RxSpringStiffnessUnits=N*m/deg  RxDampingCoefficient=0  RxDampingCoefficientUnits=N*m/(deg/s)  RxTorqueActuationMode=ComputedTorque  RxMotionActuationMode=InputMotion  RxSensePosition=off  RxSenseVelocity=off  RxSenseAcceleration=off  RxSenseTorqueForce=off  RxPositionTargetSpecify=off  RxPositionTargetPriority=High  RxPositionTargetValue=0  RxPositionTargetValueUnits=deg  RxVelocityTargetSpecify=off  RxVelocityTargetPriority=High  RxVelocityTargetValue=0  RxVelocityTargetValueUnits=deg/s  RyEquilibriumPosition=0  RyEquilibriumPositionUnits=deg  RySpringStiffness=0  RySpringStiffnessUnits=N*m/deg  RyDampingCoefficient=0  RyDampingCoefficientUnits=N*m/(deg/s)  RyTorqueActuationMode=ComputedTorque  RyMotionActuationMode=InputMotion  RySensePosition=off  RySenseVelocity=off  RySenseAcceleration=off  RySenseTorqueForce=off  RyPositionTargetSpecify=off  RyPositionTargetPriority=High  RyPositionTargetValue=0  RyPositionTargetValueUnits=deg  RyVelocityTargetSpecify=off  RyVelocityTargetPriority=High  RyVelocityTargetValue=0  RyVelocityTargetValueUnits=deg/s
      settings: SourceProductName=Simscape Multibody
  World Frame : sm_lib/Frames and Transforms/World Frame
  world : PMIOPort  Port=1  Side=Left
  Base Frame : PMIOPort  Port=2  Side=Left
  Top Platform : PMIOPort  Port=3  Side=Left
  pos : Outport
  vel : Outport  Port=2
  wires:
  Demux/1 -> [F1]
  Demux/2 -> [F2]
  Demux/3 -> [F3]
  Demux/4 -> [F4]
  Demux/5 -> [F5]
  Demux/6 -> [F6]
  [F1] -> Leg 1/1
  [F2] -> Leg 2/1
  [F3] -> Leg 3/1
  [F4] -> Leg 4/1
  [F5] -> Leg 5/1
  [F6] -> Leg 6/1
  force/1 -> Demux/1
  Leg 1/1 -> [P1]
  Leg 1/2 -> [V1]
  Leg 2/1 -> [P2]
  Leg 2/2 -> [V2]
  Leg 3/1 -> [P3]
  Leg 3/2 -> [V3]
  Leg 4/1 -> [P4]
  Leg 4/2 -> [V4]
  Leg 5/1 -> [P5]
  Leg 5/2 -> [V5]
  Leg 6/1 -> [P6]
  Leg 6/2 -> [V6]
  Mux/1 -> pos/1
  [P1] -> Mux/1
  [P2] -> Mux/2
  [P3] -> Mux/3
  [P4] -> Mux/4
  [P5] -> Mux/5
  [P6] -> Mux/6
  [V1] -> Mux1/1
  [V2] -> Mux1/2
  [V3] -> Mux1/3
  [V4] -> Mux1/4
  [V5] -> Mux1/5
  [V6] -> Mux1/6
  Mux1/1 -> vel/1
  Sine Wave Function/1 -> Simulink-PS Converter3/1
  Sine Wave Function1/1 -> Simulink-PS Converter1/1
  Clock/1 -> Sine Wave Function1/1, Sine Wave Function/1
  connections:
  Base/RConn6 -- Leg 6/LConn1
  Base/RConn5 -- Leg 5/LConn1
  Base/RConn2 -- Leg 2/LConn1
  Base/RConn1 -- Leg 1/LConn1
  Base/RConn3 -- Leg 3/LConn1
  Base/RConn4 -- Leg 4/LConn1
  Leg 1/RConn1 -- Platform/RConn1
  Leg 2/RConn1 -- Platform/RConn2
  Leg 5/RConn1 -- Platform/RConn5
  Leg 6/RConn1 -- Platform/RConn6
  Leg 3/RConn1 -- Platform/RConn3
  Leg 4/RConn1 -- Platform/RConn4
  Universal Joint/RConn1 -- Rigid Transform2/LConn1 -- Base/LConn1
  world/RConn1 -- Universal Joint/LConn1 -- World Frame/RConn1 -- Mechanism Configuration/RConn1
  Simulink-PS Converter3/RConn1 -- Universal Joint/LConn2
  Simulink-PS Converter1/RConn1 -- Universal Joint/LConn3
  Platform/LConn1 -- Top Platform/RConn1 -- Solver Configuration/RConn1
  Base Frame/RConn1 -- Rigid Transform2/RConn1

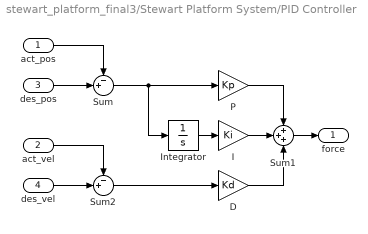
== system stewart_platform_final3/Stewart Platform System/PID Controller ==
  act_pos : Inport
  act_vel : Inport  Port=2
  des_pos : Inport  Port=3
  des_vel : Inport  Port=4
  D : Gain  Gain=Kd  SaturateOnIntegerOverflow=on  OutDataTypeStr=Inherit: Same as input  ParamDataTypeStr=Inherit: Same as input
  I : Gain  Gain=Ki  SaturateOnIntegerOverflow=on  OutDataTypeStr=Inherit: Same as input  ParamDataTypeStr=Inherit: Same as input
  Integrator : Integrator  ZeroCross=off
  P : Gain  Gain=Kp  SaturateOnIntegerOverflow=on  OutDataTypeStr=Inherit: Same as input  ParamDataTypeStr=Inherit: Same as input
  Sum : Sum  Inputs=-+|  SaturateOnIntegerOverflow=on  InputSameDT=on  OutDataTypeStr=Inherit: Same as first input
  Sum1 : Sum  Inputs=+++  SaturateOnIntegerOverflow=on  InputSameDT=on  OutDataTypeStr=Inherit: Same as first input
  Sum2 : Sum  Inputs=-+|  SaturateOnIntegerOverflow=on  InputSameDT=on  OutDataTypeStr=Inherit: Same as first input
  force : Outport
  wires:
  Sum2/1 -> D/1
  D/1 -> Sum1/3
  Integrator/1 -> I/1
  P/1 -> Sum1/1
  I/1 -> Sum1/2
  Sum/1 -> P/1, Integrator/1
  act_pos/1 -> Sum/1
  des_pos/1 -> Sum/2
  Sum1/1 -> force/1
  act_vel/1 -> Sum2/1
  des_vel/1 -> Sum2/2

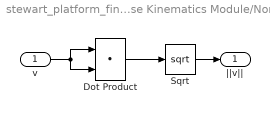
== system stewart_platform_final3/Stewart Platform System/Inverse Kinematics Module/Norm 1 ==
  v : Inport
  Dot Product : DotProduct  OutDataTypeStr=Inherit: Inherit via internal rule
  Sqrt : Sqrt  SaturateOnIntegerOverflow=on
  ||v|| : Outport
  wires:
  Dot Product/1 -> Sqrt/1
  Sqrt/1 -> ||v||/1
  v/1 -> Dot Product/1, Dot Product/2

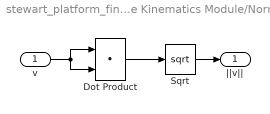
== system stewart_platform_final3/Stewart Platform System/Inverse Kinematics Module/Norm 10 ==
  v : Inport
  Dot Product : DotProduct  OutDataTypeStr=Inherit: Inherit via internal rule
  Sqrt : Sqrt  SaturateOnIntegerOverflow=on
  ||v|| : Outport
  wires:
  v/1 -> Dot Product/2, Dot Product/1
  Sqrt/1 -> ||v||/1
  Dot Product/1 -> Sqrt/1
